simulink subsystem "rss_MotoTempHiLvl2Dia"  (R2023a)
settings: Solver=VariableStepAuto  StartTime=0.0  StopTime=10.0  RelTol=1e-3
undefined symbols (not defined in the file): ENM_TYPE_FALT, Gu16_ctMotoTempHiLvl2ConfCnt_C, Gu16_ctMotoTempHiLvl2RcvyCnt_C, Gu8_tMotoTempHiLvl2ConfTrs_C, Gu8_tMotoTempHiLvl2RcvyTrs_C
libraries: vhit_control_library x1, lib_fault_definiteness x1
settings Model: Creator=xiaoqiang.yuan  LastModifiedBy=xiaoqiang.yuan

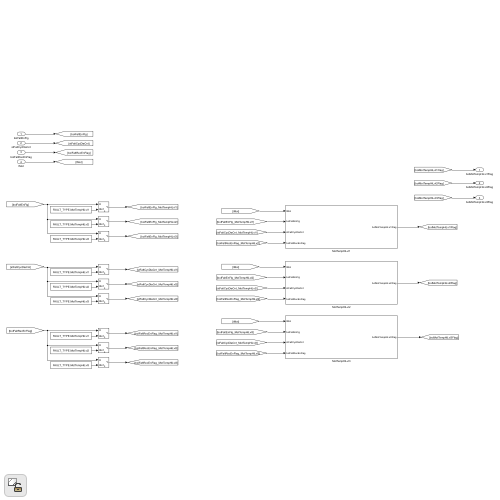
[thumbnail: Simulink's stored preview of the top-level diagram]
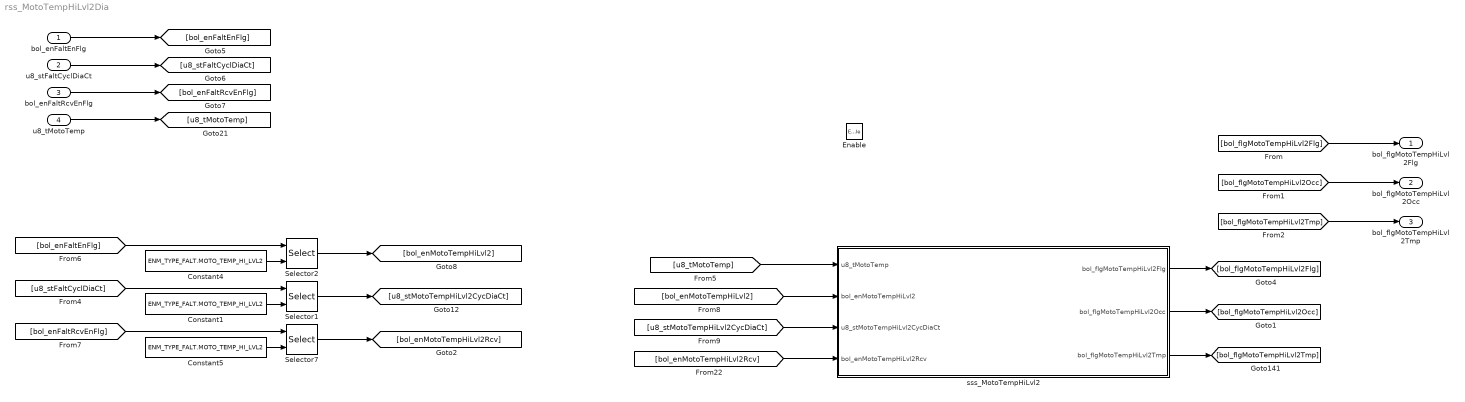
== system rss_MotoTempHiLvl2Dia ==
  bol_enFaltEnFlg : Inport  OutDataTypeStr=boolean
  u8_stFaltCyclDiaCt : Inport  Port=2  OutDataTypeStr=uint8
  bol_enFaltRcvEnFlg : Inport  Port=3  OutDataTypeStr=boolean
  u8_tMotoTemp : Inport  Port=4  OutDataTypeStr=dt_Temp_u8p0bn40
  Enable : EnablePort
  Constant1 : Constant  Value=ENM_TYPE_FALT.MOTO_TEMP_HI_LVL2
  Constant4 : Constant  Value=ENM_TYPE_FALT.MOTO_TEMP_HI_LVL2
  Constant5 : Constant  Value=ENM_TYPE_FALT.MOTO_TEMP_HI_LVL2
  Selector1 : Selector  IndexMode=Zero-based  InputPortWidth=Cdbl_numFaltDiaNum  IndexOptions=Index vector (port)  Indices=[1 3]  OutputSizes=1
  Selector2 : Selector  IndexMode=Zero-based  InputPortWidth=Cdbl_numFaltDiaNum  IndexOptions=Index vector (port)  Indices=[1 3]  OutputSizes=1
  Selector7 : Selector  IndexMode=Zero-based  InputPortWidth=Cdbl_numFaltDiaNum  IndexOptions=Index vector (port)  Indices=[1 3]  OutputSizes=1
  sss_MotoTempHiLvl2 : Subsystem
  bol_flgMotoTempHiLvl2Flg : Outport  OutDataTypeStr=boolean
  bol_flgMotoTempHiLvl2Occ : Outport  Port=2  OutDataTypeStr=boolean
  bol_flgMotoTempHiLvl2Tmp : Outport  Port=3  OutDataTypeStr=boolean
  wires:
  [bol_flgMotoTempHiLvl2Occ] -> bol_flgMotoTempHiLvl2Occ/1
  [bol_flgMotoTempHiLvl2Flg] -> bol_flgMotoTempHiLvl2Flg/1
  Selector2/1 -> [bol_enMotoTempHiLvl2]
  [bol_enMotoTempHiLvl2Rcv] -> sss_MotoTempHiLvl2/4(bol_enMotoTempHiLvl2Rcv)
  Selector7/1 -> [bol_enMotoTempHiLvl2Rcv]
  [bol_enFaltRcvEnFlg] -> Selector7/1
  Constant4/1 -> Selector2/2
  u8_tMotoTemp/1 -> [u8_tMotoTemp]
  Selector1/1 -> [u8_stMotoTempHiLvl2CycDiaCt]
  Constant1/1 -> Selector1/2
  [u8_tMotoTemp] -> sss_MotoTempHiLvl2/1(u8_tMotoTemp)
  [bol_enMotoTempHiLvl2] -> sss_MotoTempHiLvl2/2(bol_enMotoTempHiLvl2)
  [bol_enFaltEnFlg] -> Selector2/1
  u8_stFaltCyclDiaCt/1 -> [u8_stFaltCyclDiaCt]
  bol_enFaltRcvEnFlg/1 -> [bol_enFaltRcvEnFlg]
  [u8_stFaltCyclDiaCt] -> Selector1/1
  [u8_stMotoTempHiLvl2CycDiaCt] -> sss_MotoTempHiLvl2/3(u8_stMotoTempHiLvl2CycDiaCt)
  bol_enFaltEnFlg/1 -> [bol_enFaltEnFlg]
  Constant5/1 -> Selector7/2
  sss_MotoTempHiLvl2/1(bol_flgMotoTempHiLvl2Flg) -> [bol_flgMotoTempHiLvl2Flg]
  sss_MotoTempHiLvl2/2(bol_flgMotoTempHiLvl2Occ) -> [bol_flgMotoTempHiLvl2Occ]
  [bol_flgMotoTempHiLvl2Tmp] -> bol_flgMotoTempHiLvl2Tmp/1
  sss_MotoTempHiLvl2/3(bol_flgMotoTempHiLvl2Tmp) -> [bol_flgMotoTempHiLvl2Tmp]

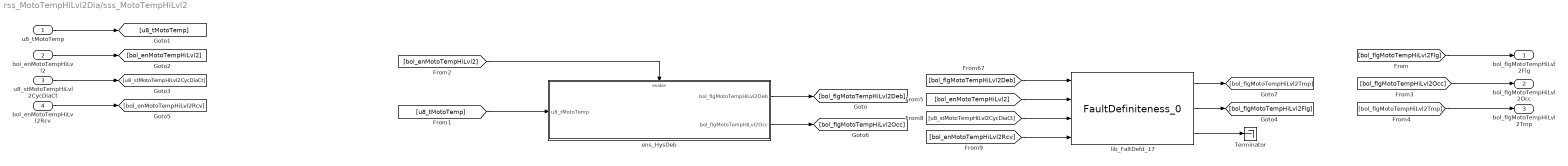
== system rss_MotoTempHiLvl2Dia/sss_MotoTempHiLvl2 ==
  u8_tMotoTemp : Inport
  bol_enMotoTempHiLvl2 : Inport  Port=2
  u8_stMotoTempHiLvl2CycDiaCt : Inport  Port=3
  bol_enMotoTempHiLvl2Rcv : Inport  Port=4
  Terminator : Terminator
  ens_HysDeb : Subsystem
  lib_FaltDefd_17 : lib_fault_definiteness/FaultDefiniteness_0  lb_FaltWaitRecvCnt=Gu16_ctMotoTempHiLvl2ConfCnt_C
  bol_flgMotoTempHiLvl2Flg : Outport
  bol_flgMotoTempHiLvl2Occ : Outport  Port=2
  bol_flgMotoTempHiLvl2Tmp : Outport  Port=3
  wires:
  [bol_flgMotoTempHiLvl2Tmp] -> bol_flgMotoTempHiLvl2Tmp/1
  [bol_flgMotoTempHiLvl2Occ] -> bol_flgMotoTempHiLvl2Occ/1
  ens_HysDeb/2(bol_flgMotoTempHiLvl2Occ) -> [bol_flgMotoTempHiLvl2Occ]
  lib_FaltDefd_17/1 -> [bol_flgMotoTempHiLvl2Tmp]
  lib_FaltDefd_17/2 -> [bol_flgMotoTempHiLvl2Flg]
  lib_FaltDefd_17/3 -> Terminator/1
  [bol_enMotoTempHiLvl2] -> ens_HysDeb/Enable
  [u8_tMotoTemp] -> ens_HysDeb/1(u8_tMotoTemp)
  ens_HysDeb/1(bol_flgMotoTempHiLvl2Deb) -> [bol_flgMotoTempHiLvl2Deb]
  bol_enMotoTempHiLvl2Rcv/1 -> [bol_enMotoTempHiLvl2Rcv]
  u8_stMotoTempHiLvl2CycDiaCt/1 -> [u8_stMotoTempHiLvl2CycDiaCt]
  bol_enMotoTempHiLvl2/1 -> [bol_enMotoTempHiLvl2]
  [bol_flgMotoTempHiLvl2Flg] -> bol_flgMotoTempHiLvl2Flg/1
  u8_tMotoTemp/1 -> [u8_tMotoTemp]
  [bol_enMotoTempHiLvl2Rcv] -> lib_FaltDefd_17/4
  [u8_stMotoTempHiLvl2CycDiaCt] -> lib_FaltDefd_17/3
  [bol_enMotoTempHiLvl2] -> lib_FaltDefd_17/2
  [bol_flgMotoTempHiLvl2Deb] -> lib_FaltDefd_17/1

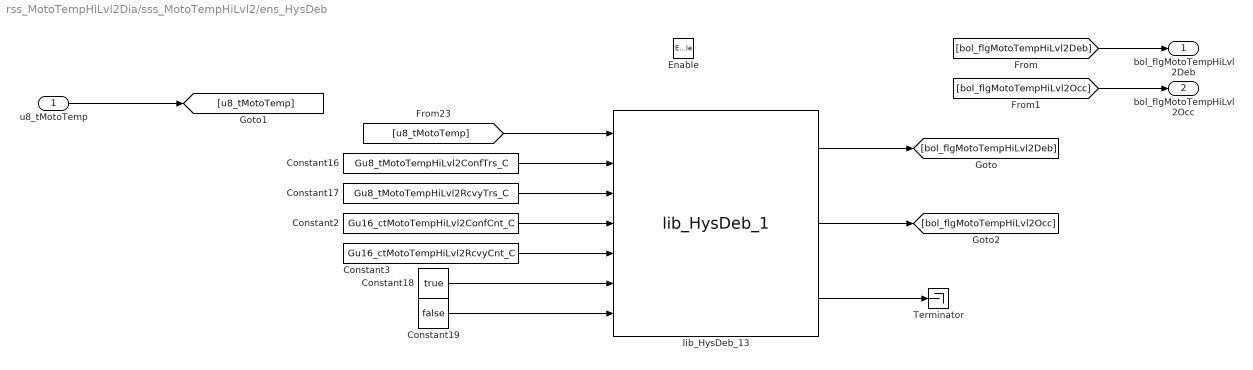
== system rss_MotoTempHiLvl2Dia/sss_MotoTempHiLvl2/ens_HysDeb ==
  u8_tMotoTemp : Inport
  Enable : EnablePort
  Constant16 : Constant  Value=Gu8_tMotoTempHiLvl2ConfTrs_C
  Constant17 : Constant  Value=Gu8_tMotoTempHiLvl2RcvyTrs_C
  Constant18 : Constant  Value=true  OutDataTypeStr=boolean
  Constant19 : Constant  Value=false  OutDataTypeStr=boolean
  Constant2 : Constant  Value=Gu16_ctMotoTempHiLvl2ConfCnt_C
  Constant3 : Constant  Value=Gu16_ctMotoTempHiLvl2RcvyCnt_C
  Terminator : Terminator
  lib_HysDeb_13 : vhit_control_library/lib_HysDeb_1  lb_parInitOutp=0
  bol_flgMotoTempHiLvl2Deb : Outport
  bol_flgMotoTempHiLvl2Occ : Outport  Port=2
  wires:
  [bol_flgMotoTempHiLvl2Occ] -> bol_flgMotoTempHiLvl2Occ/1
  lib_HysDeb_13/2 -> [bol_flgMotoTempHiLvl2Occ]
  lib_HysDeb_13/3 -> Terminator/1
  Constant3/1 -> lib_HysDeb_13/5
  Constant2/1 -> lib_HysDeb_13/4
  Constant19/1 -> lib_HysDeb_13/7
  Constant18/1 -> lib_HysDeb_13/6
  Constant17/1 -> lib_HysDeb_13/3
  Constant16/1 -> lib_HysDeb_13/2
  [u8_tMotoTemp] -> lib_HysDeb_13/1
  u8_tMotoTemp/1 -> [u8_tMotoTemp]
  [bol_flgMotoTempHiLvl2Deb] -> bol_flgMotoTempHiLvl2Deb/1
  lib_HysDeb_13/1 -> [bol_flgMotoTempHiLvl2Deb]
